simulink model "P414_1_model03_comp"  (R2021a)
settings: Solver=ode23tb  StartTime=0.0  StopTime=10  MaxStep=10/(60*24)  RelTol=1e-3
model workspace (MAT data in the model file):
  clima__A_c = 3295.16408265
  clima__A_f = 3100.53942116
  clima__G0 = [0.05; 0.00070738]
  clima__H = 7.9995824611
  clima__T0 = [287.15; 287.15; 287.15; 287.15]
  clima__T_ss = 280.150340169
  clima__alpha_c = 0.0100640347387
  clima__alpha_f = 0.0111385012129
  clima__alpha_i = 0.1
  clima__c_s = [1081 1081]
  clima__cd_c = 8736
  clima__d_c = 1.5
  clima__hour0 = 1
  clima__int_air_speed = 0.5
  clima__l_s = [0.1 0.1]
  clima__lam_s = [2.5 0.85]
  clima__minWindows = 0.299965865643
  clima__rhod_s = [2600 2500]
  clima__tau_c = 1
  crop__A_v = 2080
  crop__C = [0.01 0.001 0.01 0.01]
  crop__C_buf_max = 0.02
  crop__C_wv = 0.2
  crop__Chi_nutrients = [0.015625; 0.0104166666667; 0.00520833333333; 0.00208333333333; 0.00208333333333; 0.00104166666667; 0; 0]
  crop__N = [0; 0; 0; 0; 0; 0; 0; 0]
  crop__R = [0 0 0]
  crop__T_max_v = 40
  crop__T_max_v24 = 27
  crop__T_min_v = 6
  crop__T_min_v24 = 14
  crop__T_sum_end = 1035
  crop__T_v_start_fruit = 1100
  crop__Tsum = 0
  crop__Tv = 288
  crop__b_N_uptake = 0.5
  crop__c_fruit_g = 0.27
  crop__c_fruit_m = 2.3e-07
  crop__c_leaf_g = 0.28
  crop__c_leaf_m = 3.47e-07
  crop__c_stem_g = 0.3
  crop__c_stem_m = 1.47e-07
  crop__fraction_DM = 0.08
  crop__int_air_speed = 0.5
  crop__min_water_capacity = 0.1
  crop__plants_density = 2.1562
  crop__rg_fruit = 2e-07
  crop__rg_leaf = 9.5e-08
  crop__rg_stem = 7.4e-08
  crop__s_buforg_buf = -5000
  crop__s_max_T = 0.5793
  crop__s_max_T24 = 1.3904
  crop__s_min_T = -0.869
  crop__s_min_T24 = -1.1587
  heater__A_e = 0.0001
  heater__A_i = 0.008
  heater__T = 288
  heater__c = 5e-10
  heater__power = 60000000
  screen__Power = 100
  screen__Radthreshold = 900
  screen__beta = 2.23564167038e-14
  screen__gamma_max = 2.26308905438e-14
  screen__velocity = 0.333333333333
  subtrate__C_ws = 0.1
  subtrate__N = [0; 0; 0; 0; 0; 0; 0; 0]
  subtrate__Nmin_subs = 1e-09
  subtrate__Vmax_subs = 10
  subtrate__Vmin_subs = 0.01
  subtrate__sigma_max = 1
  subtrate__sigma_min = 1
  tomato__Cfruit0 = 0.001
  windows__AR = 19.9974923936
  windows__Power = 100
  windows__RadThreshold = 10
  windows__max_night = 10
  windows__tau = 600
values from neighbouring files (symbols this model uses):
  CO2_ppm_ext = 450    [P414_3_script_model03.m]    (also in P414_3_script_model03_compile.m = 400)
  maxvelocity = 1    [P414_3_script_model03.m]    (also in P414_3_script_model03_compile.m = 200)
  tend_crop1 = -days(t0-datetime('15-Aug-2022'))    [P414_3_script_model03.m]    (also in P414_3_script_model03_compile.m = 20)
  tend_crop2 = -days(t0-datetime('10-Dec-2022'))    [P414_3_script_model03.m]    (also in P414_3_script_model03_compile.m = 40)
  tinit_crop1 = -days(t0-datetime('16-Feb-2022'))    [P414_3_script_model03.m]    (also in P414_3_script_model03_compile.m = 1)
  tinit_crop2 = -days(t0-datetime('10-Jul-2022'))    [P414_3_script_model03.m]    (also in P414_3_script_model03_compile.m = 20)
  Tmax = 12 + 273.15    (= 285.15)    [P414_3_script_model03.m]
  today_days = floor(days(r.DateTime(end) - t0))    [P414_3_script_model03.m]    (also in P414_3_script_model03_compile.m = 5)
  Tstart = 9 + 273.15    (= 282.15)    [P414_3_script_model03.m]
  WinAR = 40    [P414_3_script_model03.m]    (also in P414_3_script_model03_compile.m = 10)
libraries: HORTISIM x15
settings Model: VariantFading=off  ParameterArgumentNames=clima__A_c,clima__A_f  OrderedModelArguments=off  Creator=djoroya  LastModifiedBy=djoroya
settings SolverCC: MaxConsecutiveMinStep=2
settings DataIOCC: SaveFormat=StructureWithTime
settings DebuggingCC: UnconnectedInputMsg=none  UnconnectedOutputMsg=none  UnconnectedLineMsg=none
settings HardwareCC: TargetBitPerLong=64  TargetBitPerPointer=64  TargetBitPerSizeT=64  TargetBitPerPtrDiffT=64  TargetLongLongMode=on  TargetIntDivRoundTo=Zero  TargetEndianess=LittleEndian  TargetWordSize=64  TargetHWDeviceType=MATLAB Host  ProdEqTarget=off
settings RTWCC: Description=Rapid Simulation Target  SystemTargetFile=rsim.tlc  TemplateMakefile=rsim_default_tmf
settings RSimTargetCC: TargetLangStandard=C99 (ISO)

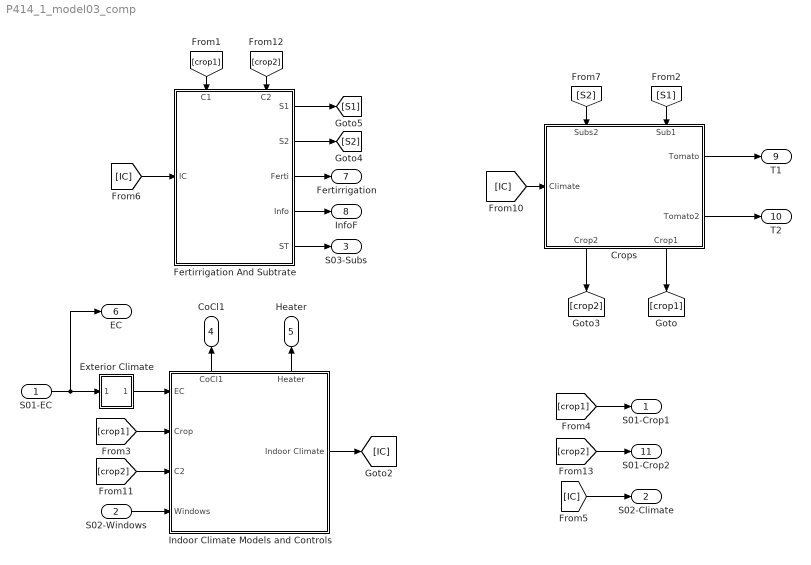
== system P414_1_model03_comp ==
  S01-EC : Inport
  S02-Windows : Inport  Port=2
  Crops : Subsystem
      settings: PortSchema="{\"entries\":[{\"content\":{\"sides\":[{\"content\":{\"connectorIds\":[\"In1\"]},\"type\":\"ConnectorPlacement.EquallySpacedRectSide\",\"uuid\":\"80596a6c-707e-446a-ab87-7a25f59fcc32\"},{\"content\":{\"connectorIds\":[\"Out1\",\"Out2\"],\"side\":\"RIGHT\"},\"type\":\"ConnectorPlacement.EquallySpacedRectSide\",\"uuid\":\"b8326ebd-de89-4eeb-b2a4-cbf566e8a818\"},{\"content\":{\"connectorIds\":[\"In2\",\"In3\"],\"side\":\"TOP\"},\"type\":\"ConnectorPlacement.EquallySpacedRectSide\",\"uuid\":\"5aa9e4b4-c649-4944-831f-92d2e7862f36\"},{\"content\":{\"connectorIds\":[\"Out3\",\"Out4\"],\"side\":\"BOTTOM\"},\"type\":\"ConnectorPlacement.EquallySpacedRectSide\",\"uuid\":\"3a07140b-9c77-4fd6-9860-89a6392cb8f1\"}]},\"type\":\"ConnectorPlacement.EquallySpacedConnector\",\"uuid\":\"ce31e92b-0c53-4f1c-a6e5-8defcbaa2f47\"}],\"packageUris\":[\"http://schema.mathworks.com/mf0/Connector/R2020b\"],\"version\":\"1.0\"}"
  Exterior Climate : Subsystem
  Fertirrigation And Subtrate : Subsystem
      settings: PortSchema="{\"entries\":[{\"content\":{\"sides\":[{\"content\":{\"connectorIds\":[\"In1\"]},\"type\":\"ConnectorPlacement.EquallySpacedRectSide\",\"uuid\":\"80596a6c-707e-446a-ab87-7a25f59fcc32\"},{\"content\":{\"connectorIds\":[\"Out1\",\"Out2\",\"Out3\",\"Out4\",\"Out5\"],\"side\":\"RIGHT\"},\"type\":\"ConnectorPlacement.EquallySpacedRectSide\",\"uuid\":\"b8326ebd-de89-4eeb-b2a4-cbf566e8a818\"},{\"content\":{\"connectorIds\":[\"In2\",\"In3\"],\"side\":\"TOP\"},\"type\":\"ConnectorPlacement.EquallySpacedRectSide\",\"uuid\":\"5aa9e4b4-c649-4944-831f-92d2e7862f36\"}]},\"type\":\"ConnectorPlacement.EquallySpacedConnector\",\"uuid\":\"ce31e92b-0c53-4f1c-a6e5-8defcbaa2f47\"}],\"packageUris\":[\"http://schema.mathworks.com/mf0/Connector/R2020b\"],\"version\":\"1.0\"}"
  Indoor Climate Models and Controls : Subsystem
      settings: PortSchema="{\"entries\":[{\"content\":{\"sides\":[{\"content\":{\"connectorIds\":[\"In1\",\"In2\",\"In3\",\"In4\"]},\"type\":\"ConnectorPlacement.EquallySpacedRectSide\",\"uuid\":\"f3cdb665-05cd-4c14-b99e-86a7cbd305f2\"},{\"content\":{\"connectorIds\":[\"Out1\"],\"side\":\"RIGHT\"},\"type\":\"ConnectorPlacement.EquallySpacedRectSide\",\"uuid\":\"ae9c6689-db0e-4adc-94c4-95f30f4a2385\"},{\"content\":{\"connectorIds\":[\"Out2\",\"Out3\"],\"side\":\"TOP\"},\"type\":\"ConnectorPlacement.EquallySpacedRectSide\",\"uuid\":\"b06e03f0-9ac9-40cc-8ad1-aa848145a491\"}]},\"type\":\"ConnectorPlacement.EquallySpacedConnector\",\"uuid\":\"03211f4f-961e-418c-be17-aa45c1620fb4\"}],\"packageUris\":[\"http://schema.mathworks.com/mf0/Connector/R2020b\"],\"version\":\"1.0\"}"
  S01-Crop1 : Outport
  S02-Climate : Outport  Port=2
  S03-Subs : Outport  Port=3
  CoCl1 : Outport  Port=4
  Heater : Outport  Port=5
  EC : Outport  Port=6
  Fertirrigation : Outport  Port=7
  InfoF : Outport  Port=8
  T1 : Outport  Port=9
  T2 : Outport  Port=10
  S01-Crop2 : Outport  Port=11
  wires:
  Exterior Climate/1(EC) -> Indoor Climate Models and Controls/1(EC)
  [crop1] -> Indoor Climate Models and Controls/2(Crop)
  S01-EC/1 -> EC/1, Exterior Climate/1(In1)
  [IC] -> S02-Climate/1
  [crop1] -> S01-Crop1/1
  Indoor Climate Models and Controls/2(CoCl1) -> CoCl1/1
  S02-Windows/1 -> Indoor Climate Models and Controls/4(Windows)
  Indoor Climate Models and Controls/3(Heater) -> Heater/1
  Indoor Climate Models and Controls/1(Indoor Climate) -> [IC]
  [crop1] -> Fertirrigation And Subtrate/2(C1)
  [crop2] -> Fertirrigation And Subtrate/3(C2)
  [IC] -> Fertirrigation And Subtrate/1(IC)
  Fertirrigation And Subtrate/1(S1) -> [S1]
  Fertirrigation And Subtrate/2(S2) -> [S2]
  Fertirrigation And Subtrate/3(Ferti) -> Fertirrigation/1
  Fertirrigation And Subtrate/4(Info) -> InfoF/1
  [crop2] -> Indoor Climate Models and Controls/3(C2)
  [crop2] -> S01-Crop2/1
  [S1] -> Crops/3(Sub1)
  [IC] -> Crops/1(Climate)
  [S2] -> Crops/2(Subs2)
  Crops/4(Crop1) -> [crop1]
  Crops/1(Tomato) -> T1/1
  Crops/3(Crop2) -> [crop2]
  Crops/2(Tomato2) -> T2/1
  Fertirrigation And Subtrate/5(ST) -> S03-Subs/1

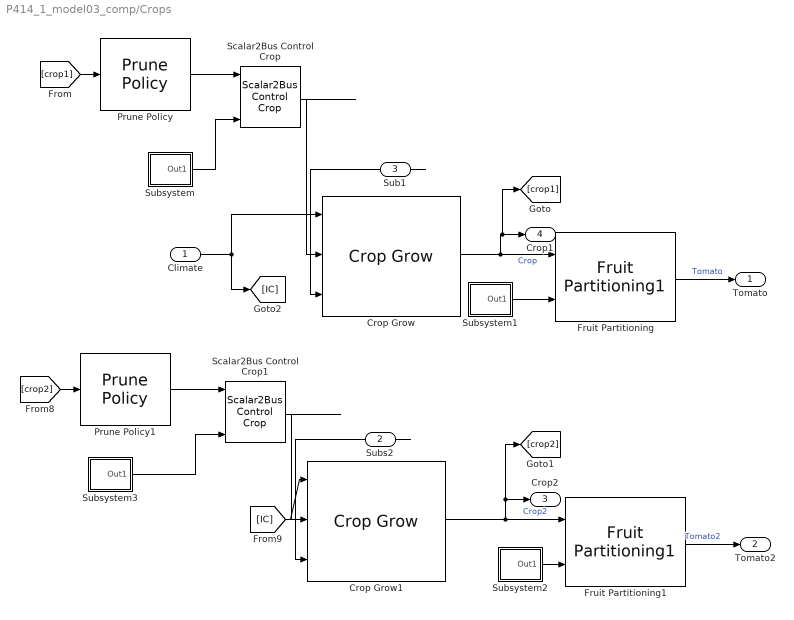
== system P414_1_model03_comp/Crops ==
  Climate : Inport
  Subs2 : Inport  Port=2
  Sub1 : Inport  Port=3
  Crop Grow : HORTISIM/Horticulture/Models/Crop Grow  Chi_nutrients=crop__Chi_nutrients  A_v=crop__A_v  plants_density=crop__plants_density  fraction_DM=crop__fraction_DM  min_water_capacity=crop__min_water_capacity  C_buf_max=crop__C_buf_max  T_v_start_fruit=crop__T_v_start_fruit  int_air_speed=crop__int_air_speed  b_N_uptake=crop__b_N_uptake  Tv=crop__Tv  C=crop__C  R=crop__R  Tsum=crop__Tsum  C_wv=crop__C_wv  N=crop__N  rg_fruit=crop__rg_fruit  c_fruit_m=crop__c_fruit_m  c_fruit_g=crop__c_fruit_g  rg_leaf=crop__rg_leaf  c_leaf_m=crop__c_leaf_m  c_leaf_g=crop__c_leaf_g  rg_stem=crop__rg_stem  c_stem_m=crop__c_stem_m  c_stem_g=crop__c_stem_g  VelocityAbsortion=crop__VelocityAbsortion  T_max_v=crop__T_max_v  s_max_T=crop__s_max_T  s_min_T=crop__s_min_T  s_buforg_buf=crop__s_buforg_buf  T_sum_end=crop__T_sum_end  T_max_v24=crop__T_max_v24  T_min_v24=crop__T_min_v24  s_min_T24=crop__s_min_T24  s_max_T24=crop__s_max_T24  T_min_v=crop__T_min_v
      settings: SourceProductName=Horti Simulator
  Crop Grow1 : HORTISIM/Horticulture/Models/Crop Grow  Chi_nutrients=crop__Chi_nutrients  A_v=crop__A_v  plants_density=crop__plants_density  fraction_DM=crop__fraction_DM  min_water_capacity=crop__min_water_capacity  C_buf_max=crop__C_buf_max  T_v_start_fruit=crop__T_v_start_fruit  int_air_speed=crop__int_air_speed  b_N_uptake=crop__b_N_uptake  Tv=crop__Tv  C=crop__C  R=crop__R  Tsum=crop__Tsum  C_wv=crop__C_wv  N=crop__N  rg_fruit=crop__rg_fruit  c_fruit_m=crop__c_fruit_m  c_fruit_g=crop__c_fruit_g  rg_leaf=crop__rg_leaf  c_leaf_m=crop__c_leaf_m  c_leaf_g=crop__c_leaf_g  rg_stem=crop__rg_stem  c_stem_m=crop__c_stem_m  c_stem_g=crop__c_stem_g  VelocityAbsortion=crop__VelocityAbsortion  T_max_v=crop__T_max_v  s_max_T=crop__s_max_T  s_min_T=crop__s_min_T  s_buforg_buf=crop__s_buforg_buf  T_sum_end=crop__T_sum_end  T_max_v24=crop__T_max_v24  T_min_v24=crop__T_min_v24  s_min_T24=crop__s_min_T24  s_max_T24=crop__s_max_T24  T_min_v=crop__T_min_v
      settings: SourceProductName=Horti Simulator
  Fruit Partitioning : HORTISIM/Horticulture/Models/Fruit Partitioning1  Cfruit0=1e-3
      settings: SourceProductName=Horti Simulator
  Fruit Partitioning1 : HORTISIM/Horticulture/Models/Fruit Partitioning1  Cfruit0=tomato__Cfruit0
      settings: SourceProductName=Horti Simulator
  Prune Policy : HORTISIM/Horticulture/Controls/Prune Policy  SystemSampleTime=-1  VariantActivationTime=update diagram  Latency=0  AutoFrameSizeCalculation=off
      settings: SourceProductName=Horti Simulator
  Prune Policy1 : HORTISIM/Horticulture/Controls/Prune Policy  SystemSampleTime=-1  VariantActivationTime=update diagram  Latency=0  AutoFrameSizeCalculation=off
      settings: SourceProductName=Horti Simulator
  Scalar2Bus Control Crop : HORTISIM/Other  Functions/Scalar2Bus Control Crop  SystemSampleTime=-1  VariantActivationTime=update diagram  Latency=0  AutoFrameSizeCalculation=off
      settings: SourceProductName=Horti Simulator
  Scalar2Bus Control Crop1 : HORTISIM/Other  Functions/Scalar2Bus Control Crop  SystemSampleTime=-1  VariantActivationTime=update diagram  Latency=0  AutoFrameSizeCalculation=off
      settings: SourceProductName=Horti Simulator
  Subsystem : Subsystem  mask{tinit=tinit_crop1, tend=tend_crop1}
  Subsystem1 : Subsystem  mask{tinit=tinit_crop1, tend=tend_crop1}
  Subsystem2 : Subsystem  mask{tinit=tinit_crop2, tend=tend_crop2}
  Subsystem3 : Subsystem  mask{tinit=tinit_crop2, tend=tend_crop2}
  Tomato : Outport
  Tomato2 : Outport  Port=2
  Crop2 : Outport  Port=3
  Crop1 : Outport  Port=4
  wires:
  Subs2/1 -> Crop Grow1/3
  Fruit Partitioning/1 -> Tomato/1  "Tomato"
  Scalar2Bus Control Crop1/1 -> Crop Grow1/2
  Sub1/1 -> Crop Grow/3
  Subsystem/1(Out1) -> Scalar2Bus Control Crop/4
  [IC] -> Crop Grow1/1
  [crop2] -> Prune Policy1/1
  Crop Grow1/1 -> [crop2], Crop2/1, Fruit Partitioning1/1  "Crop2"
  Fruit Partitioning1/1 -> Tomato2/1  "Tomato2"
  Subsystem1/1(Out1) -> Fruit Partitioning/2
  Prune Policy/1 -> Scalar2Bus Control Crop/1
  Subsystem2/1(Out1) -> Fruit Partitioning1/2
  [crop1] -> Prune Policy/1
  Subsystem3/1(Out1) -> Scalar2Bus Control Crop1/4
  Crop Grow/1 -> [crop1], Crop1/1, Fruit Partitioning/1  "Crop"
  Scalar2Bus Control Crop/1 -> Crop Grow/2
  Climate/1 -> [IC], Crop Grow/1
  Prune Policy1/1 -> Scalar2Bus Control Crop1/1

== system P414_1_model03_comp/Exterior Climate ==
  In1 : Inport
  CO2 ppm : Constant  Value=CO2_ppm_ext
  Demux : Demux
  Scalar2Bus Exterior Climate : Subsystem
  EC : Outport
  wires:
  Demux/3 -> Scalar2Bus Exterior Climate/3(Wind)
  Demux/2 -> Scalar2Bus Exterior Climate/2(Radiation)
  Scalar2Bus Exterior Climate/1(EC) -> EC/1
  Demux/1 -> Scalar2Bus Exterior Climate/1(Temperature)
  Demux/4 -> Scalar2Bus Exterior Climate/4(Humidity)
  In1/1 -> Demux/1
  CO2 ppm/1 -> Scalar2Bus Exterior Climate/5(CO2)

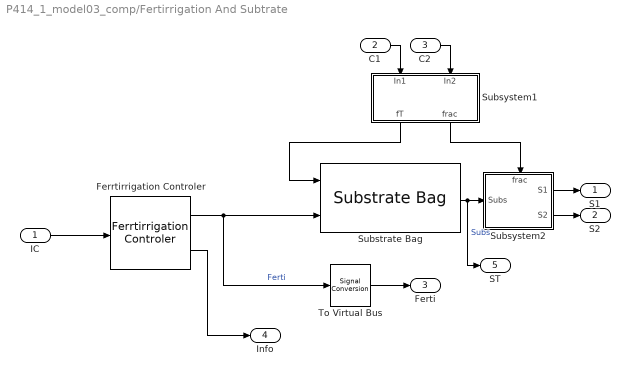
== system P414_1_model03_comp/Fertirrigation And Subtrate ==
  IC : Inport
  C1 : Inport  Port=2
  C2 : Inport  Port=3
  Ferrtirrigation Controler : HORTISIM/Horticulture/Controls/Ferrtirrigation  Controler  hour0=irrigation__hour0  IrrigationFlow=irrigation__IrrigationFlow  Xnutrients=irrigation__Xnutrients  percent_irrigation=irrigation__percent_irrigation  Irrigation_jules_to_hours=irrigation__Irrigation_jules_to_hours
      settings: SourceProductName=Horti Simulator
  Substrate Bag : HORTISIM/Horticulture/Models/Substrate Bag  Vmax_subs=subtrate__Vmax_subs  Vmin_subs=subtrate__Vmin_subs  Nmin_subs=subtrate__Nmin_subs  C_ws=subtrate__C_ws  N=subtrate__N  DraingeConst=subtrate__DraingeConst  sigma_max=subtrate__sigma_max  sigma_min=subtrate__sigma_min
      settings: SourceProductName=Horti Simulator
  Subsystem1 : Subsystem
  Subsystem2 : Subsystem
      settings: PortSchema="{\"entries\":[{\"content\":{\"sides\":[{\"content\":{\"connectorIds\":[\"In1\"]},\"type\":\"ConnectorPlacement.EquallySpacedRectSide\",\"uuid\":\"526c2ba0-7984-4a67-b75e-815cf79b4473\"},{\"content\":{\"connectorIds\":[\"Out1\",\"Out2\"],\"side\":\"RIGHT\"},\"type\":\"ConnectorPlacement.EquallySpacedRectSide\",\"uuid\":\"1f428ce7-4be7-4b4c-9b6b-ebbf12a2ebe7\"},{\"content\":{\"connectorIds\":[\"In2\"],\"side\":\"TOP\"},\"type\":\"ConnectorPlacement.EquallySpacedRectSide\",\"uuid\":\"5866ee80-50d2-4205-943e-212db577b0a0\"}]},\"type\":\"ConnectorPlacement.EquallySpacedConnector\",\"uuid\":\"0f7aadc1-005b-462a-894f-416c66164dac\"}],\"packageUris\":[\"http://schema.mathworks.com/mf0/Connector/R2020b\"],\"version\":\"1.0\"}"
  To Virtual Bus : SignalConversion  ConversionOutput=Virtual bus  OverrideOpt=off
  S1 : Outport
  S2 : Outport  Port=2
  Ferti : Outport  Port=3
  Info : Outport  Port=4
  ST : Outport  Port=5
  wires:
  C2/1 -> Subsystem1/2(In2)
  Subsystem1/2(frac) -> Subsystem2/2(frac)
  Ferrtirrigation Controler/1 -> Substrate Bag/2, To Virtual Bus/1  "Ferti"
  Subsystem2/1(S1) -> S1/1
  C1/1 -> Subsystem1/1(In1)
  Ferrtirrigation Controler/2 -> Info/1
  Subsystem2/2(S2) -> S2/1
  IC/1 -> Ferrtirrigation Controler/1
  To Virtual Bus/1 -> Ferti/1
  Substrate Bag/1 -> ST/1, Subsystem2/1(Subs)  "Subs"
  Subsystem1/1(fT) -> Substrate Bag/1

== system P414_1_model03_comp/Indoor Climate Models and Controls ==
  EC : Inport
  Crop : Inport  Port=2
  C2 : Inport  Port=3
  Windows : Inport  Port=4
  Climate Model : HORTISIM/Climate/Models/Climate Model  hour0=clima__hour0  G0=clima__G0  T0=clima__T0  H=clima__H  A_f=clima__A_f  A_c=clima__A_c  minWindows=clima__minWindows  lam_s=clima__lam_s  c_s=clima__c_s  l_s=clima__l_s  rhod_s=clima__rhod_s  int_air_speed=clima__int_air_speed  alpha_i=clima__alpha_i  alpha_c=clima__alpha_c  tau_c=clima__tau_c  alpha_f=clima__alpha_f  d_c=clima__d_c  cd_c=clima__cd_c  T_ss=clima__T_ss
      settings: SourceProductName=Horti Simulator
  Control System : Subsystem
      settings: PortSchema="{\"entries\":[{\"content\":{\"sides\":[{\"content\":{\"connectorIds\":[\"In1\",\"In2\",\"In3\",\"In4\"]},\"type\":\"ConnectorPlacement.EquallySpacedRectSide\",\"uuid\":\"7d0146e2-a53b-49ab-a7f4-04cd7ef00b9a\"},{\"content\":{\"connectorIds\":[\"Out1\",\"Out2\"],\"side\":\"RIGHT\"},\"type\":\"ConnectorPlacement.EquallySpacedRectSide\",\"uuid\":\"fee587e2-4b5c-4140-8904-07609d427593\"},{\"content\":{\"connectorIds\":[],\"side\":\"TOP\"},\"type\":\"ConnectorPlacement.EquallySpacedRectSide\",\"uuid\":\"52e767bc-1595-40ac-996f-44c9eedd0a08\"},{\"content\":{\"connectorIds\":[\"Out3\",\"In5\"],\"side\":\"BOTTOM\"},\"type\":\"ConnectorPlacement.EquallySpacedRectSide\",\"uuid\":\"c629db5c-cfe6-4bd1-aeb9-7fba46dde396\"}]},\"type\":\"ConnectorPlacement.EquallySpacedConnector\",\"uuid\":\"268fde01-3c08-4d62-bfbb-fc94284c5cdd\"}],\"packageUris\":[\"http://schema.mathworks.com/mf0/Connector/R2020b\"],\"version\":\"1.0\"}"
  Indoor Climate : Outport
  CoCl1 : Outport  Port=2
  Heater : Outport  Port=3
  wires:
  Climate Model/1 -> Control System/2(IC), Indoor Climate/1  "Indoor Climate"
  Control System/2(CoCl1) -> Climate Model/2, CoCl1/1  "Control"
  Control System/1(Ext) -> Climate Model/1
  EC/1 -> Climate Model/3, Control System/5(EC)
  Crop/1 -> Control System/3(C1)
  Windows/1 -> Control System/1(Windows)
  Control System/3(Heater) -> Heater/1
  C2/1 -> Control System/4(C2)

== system P414_1_model03_comp/Crops/Subsystem ==
  Clock : Clock
  Constant : Constant  Value=tinit
  Constant1 : Constant  Value=tend
  If : If  NumInputs=3  IfExpression=(u1>u2)&(u1<u3)
  If Action Subsystem : Subsystem  TreatAsAtomicUnit=on
  If Action Subsystem1 : Subsystem  TreatAsAtomicUnit=on
  Merge : Merge
  Out1 : Outport
  wires:
  Clock/1 -> If/1
  Constant/1 -> If/2
  Constant1/1 -> If/3
  If/1 -> If Action Subsystem/Action
  If/2 -> If Action Subsystem1/Action
  If Action Subsystem/1(Out1) -> Merge/1
  If Action Subsystem1/1(Out1) -> Merge/2
  Merge/1 -> Out1/1

== system P414_1_model03_comp/Crops/Subsystem1 ==
  Clock : Clock
  Constant : Constant  Value=tinit
  Constant1 : Constant  Value=tend
  If : If  NumInputs=3  IfExpression=(u1>u2)&(u1<u3)
  If Action Subsystem : Subsystem  TreatAsAtomicUnit=on
  If Action Subsystem1 : Subsystem  TreatAsAtomicUnit=on
  Merge : Merge
  Out1 : Outport
  wires:
  Clock/1 -> If/1
  Constant/1 -> If/2
  Constant1/1 -> If/3
  If/1 -> If Action Subsystem/Action
  If/2 -> If Action Subsystem1/Action
  If Action Subsystem/1(Out1) -> Merge/1
  If Action Subsystem1/1(Out1) -> Merge/2
  Merge/1 -> Out1/1

== system P414_1_model03_comp/Crops/Subsystem2 ==
  Clock : Clock
  Constant : Constant  Value=tinit
  Constant1 : Constant  Value=tend
  If : If  NumInputs=3  IfExpression=(u1>u2)&(u1<u3)
  If Action Subsystem : Subsystem  TreatAsAtomicUnit=on
  If Action Subsystem1 : Subsystem  TreatAsAtomicUnit=on
  Merge : Merge
  Out1 : Outport
  wires:
  Clock/1 -> If/1
  Constant/1 -> If/2
  Constant1/1 -> If/3
  If/1 -> If Action Subsystem/Action
  If/2 -> If Action Subsystem1/Action
  If Action Subsystem/1(Out1) -> Merge/1
  If Action Subsystem1/1(Out1) -> Merge/2
  Merge/1 -> Out1/1

== system P414_1_model03_comp/Crops/Subsystem3 ==
  Clock : Clock
  Constant : Constant  Value=tinit
  Constant1 : Constant  Value=tend
  If : If  NumInputs=3  IfExpression=(u1>u2)&(u1<u3)
  If Action Subsystem : Subsystem  TreatAsAtomicUnit=on
  If Action Subsystem1 : Subsystem  TreatAsAtomicUnit=on
  Merge : Merge
  Out1 : Outport
  wires:
  Clock/1 -> If/1
  Constant/1 -> If/2
  Constant1/1 -> If/3
  If/1 -> If Action Subsystem/Action
  If/2 -> If Action Subsystem1/Action
  If Action Subsystem/1(Out1) -> Merge/1
  If Action Subsystem1/1(Out1) -> Merge/2
  Merge/1 -> Out1/1

== system P414_1_model03_comp/Exterior Climate/Scalar2Bus Exterior Climate ==
  Temperature : Inport
  Radiation : Inport  Port=2
  Wind : Inport  Port=3
  Humidity : Inport  Port=4
  CO2 : Inport  Port=5
  Bus Creator : BusCreator  Inputs=5
  EC : Outport
  wires:
  Humidity/1 -> Bus Creator/3  "HR"
  Wind/1 -> Bus Creator/4  "Wind"
  Temperature/1 -> Bus Creator/1  "Temp"
  Bus Creator/1 -> EC/1
  Radiation/1 -> Bus Creator/2  "Rad"
  CO2/1 -> Bus Creator/5  "Cppm"

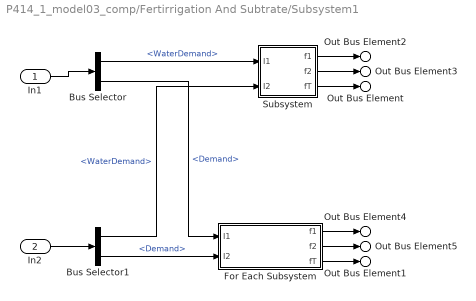
== system P414_1_model03_comp/Fertirrigation And Subtrate/Subsystem1 ==
  In1 : Inport
  In2 : Inport  Port=2
  Bus Selector : BusSelector  OutputSignals=Water.WaterFlows.WaterDemand,Nutrients.Demand
  Bus Selector1 : BusSelector  OutputSignals=Water.WaterFlows.WaterDemand,Nutrients.Demand
  For Each Subsystem : Subsystem  TreatAsAtomicUnit=on
  Subsystem : Subsystem
  Out Bus Element1 : Outport  PortName=fT  Element=Nutrients.Demand
  Out Bus Element : Outport  PortName=fT  Element=Water.WaterFlows.WaterDemand
  Out Bus Element2 : Outport  Port=2  PortName=frac  Element=water.f1
  Out Bus Element3 : Outport  Port=2  PortName=frac  Element=water.f2
  Out Bus Element4 : Outport  Port=2  PortName=frac  Element=nutrients.f1
  Out Bus Element5 : Outport  Port=2  PortName=frac  Element=nutrients.f2
  wires:
  In1/1 -> Bus Selector/1
  In2/1 -> Bus Selector1/1
  Bus Selector1/1 -> Subsystem/2(I2)  "<WaterDemand>"
  Bus Selector/1 -> Subsystem/1(I1)  "<WaterDemand>"
  Subsystem/3(fT) -> Out Bus Element/1
  Subsystem/1(f1) -> Out Bus Element2/1
  Subsystem/2(f2) -> Out Bus Element3/1
  Bus Selector/2 -> For Each Subsystem/1(I1)  "<Demand>"
  Bus Selector1/2 -> For Each Subsystem/2(I2)  "<Demand>"
  For Each Subsystem/3(fT) -> Out Bus Element1/1
  For Each Subsystem/2(f2) -> Out Bus Element5/1
  For Each Subsystem/1(f1) -> Out Bus Element4/1

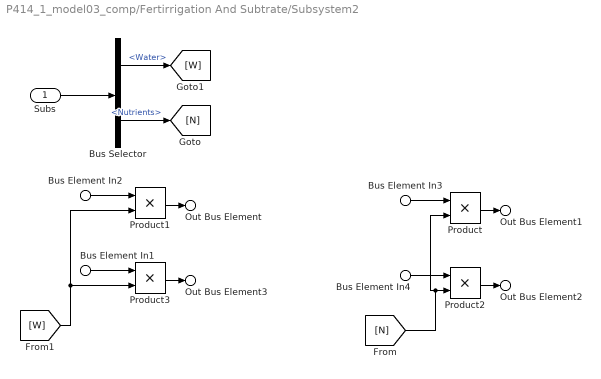
== system P414_1_model03_comp/Fertirrigation And Subtrate/Subsystem2 ==
  Subs : Inport
  Bus Element In2 : Inport  Port=2  PortName=frac  Element=water.f1
  Bus Element In1 : Inport  Port=2  PortName=frac  Element=water.f2
  Bus Element In3 : Inport  Port=2  PortName=frac  Element=nutrients.f1
  Bus Element In4 : Inport  Port=2  PortName=frac  Element=nutrients.f2
  Bus Selector : BusSelector  OutputSignals=Uptake.Water,Uptake.Nutrients
  Product{,1..3} (4 alike) : Product
  Out Bus Element : Outport  PortName=S1  Element=Uptake.Water
  Out Bus Element1 : Outport  PortName=S1  Element=Uptake.Nutrients
  Out Bus Element3 : Outport  Port=2  PortName=S2  Element=Uptake.Water
  Out Bus Element2 : Outport  Port=2  PortName=S2  Element=Uptake.Nutrients
  wires:
  Subs/1 -> Bus Selector/1
  Bus Selector/1 -> [W]  "<Water>"
  Bus Selector/2 -> [N]  "<Nutrients>"
  Bus Element In3/1 -> Product/1
  Bus Element In2/1 -> Product1/1
  Bus Element In4/1 -> Product2/1
  [N] -> Product/2, Product2/2
  Bus Element In1/1 -> Product3/1
  [W] -> Product3/2, Product1/2
  Product1/1 -> Out Bus Element/1
  Product3/1 -> Out Bus Element3/1
  Product/1 -> Out Bus Element1/1
  Product2/1 -> Out Bus Element2/1

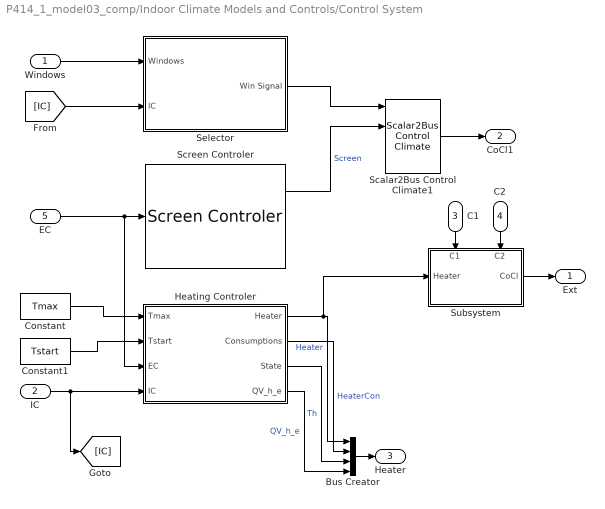
== system P414_1_model03_comp/Indoor Climate Models and Controls/Control System ==
  Windows : Inport
  IC : Inport  Port=2
  C1 : Inport  Port=3
  C2 : Inport  Port=4
  EC : Inport  Port=5
  Bus Creator : BusCreator  Inputs=4
  Constant : Constant  Value=Tmax
  Constant1 : Constant  Value=Tstart
  Heating Controler : Subsystem  AncestorBlock=HORTISIM/Climate/Controls/Heating Controler  mask{T=heater__T, power=heater__power, A_e=heater__A_e, A_i=heater__A_i, c=heater__c}
      mask DialogControl InitialCondition Prompt: Initial Condition
      mask DialogControl Parameters Prompt: Parameters
      mask Display: image('$imagefile'); % Use "Edit Image" on toolstrip to change.
  Scalar2Bus Control Climate1 : HORTISIM/Other  Functions/Scalar2Bus  Control Climate  SystemSampleTime=-1  VariantActivationTime=update diagram  Latency=0  AutoFrameSizeCalculation=off
      settings: SourceProductName=Horti Simulator
  Screen Controler : HORTISIM/Climate/Controls/Screen Controler  Radthreshold=200  velocity=0.33333  Power=0  gamma_max=0.3  beta=0.1
      settings: SourceProductName=Horti Simulator
  Selector : Subsystem
  Subsystem : Subsystem
      settings: PortSchema="{\"entries\":[{\"content\":{\"sides\":[{\"content\":{\"connectorIds\":[\"In1\"]},\"type\":\"ConnectorPlacement.EquallySpacedRectSide\",\"uuid\":\"d19974ff-f02b-4de0-b9d2-af7ff1541749\"},{\"content\":{\"connectorIds\":[\"Out1\"],\"side\":\"RIGHT\"},\"type\":\"ConnectorPlacement.EquallySpacedRectSide\",\"uuid\":\"996386bc-d441-4074-8822-a847efaf7161\"},{\"content\":{\"connectorIds\":[\"In2\",\"In3\"],\"side\":\"TOP\"},\"type\":\"ConnectorPlacement.EquallySpacedRectSide\",\"uuid\":\"19980254-f226-445c-8822-1dc223142f79\"}]},\"type\":\"ConnectorPlacement.EquallySpacedConnector\",\"uuid\":\"a52359a0-275e-4596-8c51-69b7f984311f\"}],\"packageUris\":[\"http://schema.mathworks.com/mf0/Connector/R2020b\"],\"version\":\"1.0\"}"
  Ext : Outport
  CoCl1 : Outport  Port=2
  Heater : Outport  Port=3
  wires:
  EC/1 -> Heating Controler/3(EC), Screen Controler/1
  Constant1/1 -> Heating Controler/2(Tstart)
  Constant/1 -> Heating Controler/1(Tmax)
  Scalar2Bus Control Climate1/1 -> CoCl1/1
  Screen Controler/1 -> Scalar2Bus Control Climate1/2  "Screen"
  IC/1 -> [IC], Heating Controler/4(IC)
  Heating Controler/1(Heater) -> Subsystem/1(Heater), Bus Creator/1  "Heater"
  Heating Controler/2(Consumptions) -> Bus Creator/2  "HeaterCon"
  Heating Controler/3(State) -> Bus Creator/3  "Th"
  Bus Creator/1 -> Heater/1
  Windows/1 -> Selector/1(Windows)
  Selector/1(Win Signal) -> Scalar2Bus Control Climate1/1
  [IC] -> Selector/2(IC)
  Heating Controler/4(QV_h_e) -> Bus Creator/4  "QV_h_e"
  C2/1 -> Subsystem/3(C2)
  C1/1 -> Subsystem/2(C1)
  Subsystem/1(CoCl) -> Ext/1

== system P414_1_model03_comp/Crops/Subsystem/If Action Subsystem ==
  Action Port : ActionPort  ActionPortLabel=if((u1>u2)&(u1<u3))
  Constant : Constant
  Out1 : Outport
  wires:
  Constant/1 -> Out1/1

== system P414_1_model03_comp/Crops/Subsystem/If Action Subsystem1 ==
  Action Port : ActionPort  ActionPortLabel=else
  Constant : Constant  Value=0
  Out1 : Outport
  wires:
  Constant/1 -> Out1/1

== system P414_1_model03_comp/Crops/Subsystem1/If Action Subsystem ==
  Action Port : ActionPort  ActionPortLabel=if((u1>u2)&(u1<u3))
  Constant : Constant
  Out1 : Outport
  wires:
  Constant/1 -> Out1/1

== system P414_1_model03_comp/Crops/Subsystem1/If Action Subsystem1 ==
  Action Port : ActionPort  ActionPortLabel=else
  Constant : Constant  Value=0
  Out1 : Outport
  wires:
  Constant/1 -> Out1/1

== system P414_1_model03_comp/Crops/Subsystem2/If Action Subsystem ==
  Action Port : ActionPort  ActionPortLabel=if((u1>u2)&(u1<u3))
  Constant : Constant
  Out1 : Outport
  wires:
  Constant/1 -> Out1/1

== system P414_1_model03_comp/Crops/Subsystem2/If Action Subsystem1 ==
  Action Port : ActionPort  ActionPortLabel=else
  Constant : Constant  Value=0
  Out1 : Outport
  wires:
  Constant/1 -> Out1/1

== system P414_1_model03_comp/Crops/Subsystem3/If Action Subsystem ==
  Action Port : ActionPort  ActionPortLabel=if((u1>u2)&(u1<u3))
  Constant : Constant
  Out1 : Outport
  wires:
  Constant/1 -> Out1/1

== system P414_1_model03_comp/Crops/Subsystem3/If Action Subsystem1 ==
  Action Port : ActionPort  ActionPortLabel=else
  Constant : Constant  Value=0
  Out1 : Outport
  wires:
  Constant/1 -> Out1/1

== system P414_1_model03_comp/Fertirrigation And Subtrate/Subsystem1/For Each Subsystem ==
  I1 : Inport  Partition=on  PartitionDimension=1  PartitionWidth=1  PartitionOffset=0
  I2 : Inport  Port=2  Partition=on  PartitionDimension=1  PartitionWidth=1  PartitionOffset=0
  For Each : ForEach  DisableCoverage=on
  Subsystem : Subsystem
  f1 : Outport  ConcatenationDimension=1
  f2 : Outport  Port=2  ConcatenationDimension=1
  fT : Outport  Port=3  ConcatenationDimension=1
  wires:
  I2/1 -> Subsystem/2(I2)
  I1/1 -> Subsystem/1(I1)
  Subsystem/3(fT) -> fT/1
  Subsystem/2(f2) -> f2/1
  Subsystem/1(f1) -> f1/1

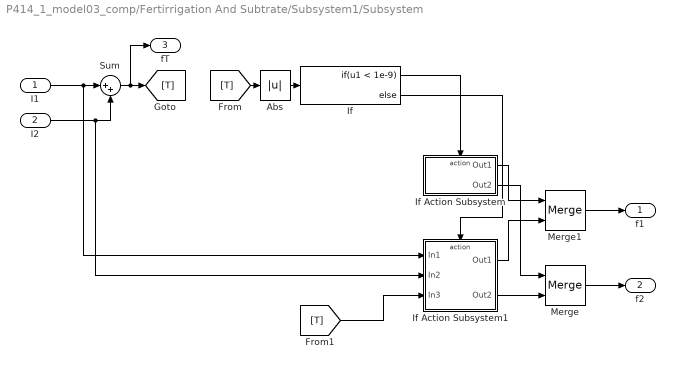
== system P414_1_model03_comp/Fertirrigation And Subtrate/Subsystem1/Subsystem ==
  I1 : Inport
  I2 : Inport  Port=2
  Abs : Abs  ZeroCross=off
  If : If  IfExpression=u1 < 1e-9  ZeroCross=off
  If Action Subsystem : Subsystem  TreatAsAtomicUnit=on
  If Action Subsystem1 : Subsystem  TreatAsAtomicUnit=on
  Merge : Merge
  Merge1 : Merge
  Sum : Sum  Inputs=|++
  f1 : Outport
  f2 : Outport  Port=2
  fT : Outport  Port=3
  wires:
  I1/1 -> If Action Subsystem1/1(In1), Sum/1
  I2/1 -> If Action Subsystem1/2(In2), Sum/2
  Sum/1 -> fT/1, [T]
  If/1 -> If Action Subsystem/Action
  If/2 -> If Action Subsystem1/Action
  [T] -> If Action Subsystem1/3(In3)
  If Action Subsystem/2(Out2) -> Merge/1
  If Action Subsystem1/2(Out2) -> Merge/2
  Merge/1 -> f2/1
  Merge1/1 -> f1/1
  If Action Subsystem1/1(Out1) -> Merge1/2
  If Action Subsystem/1(Out1) -> Merge1/1
  Abs/1 -> If/1
  [T] -> Abs/1

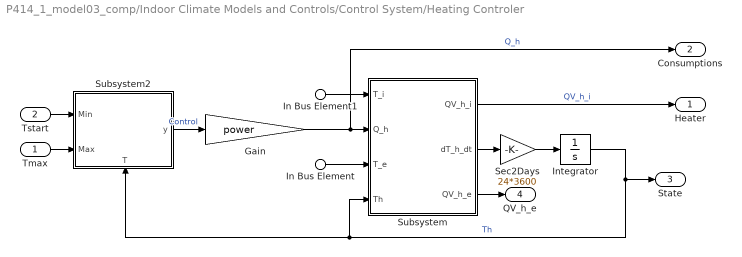
== system P414_1_model03_comp/Indoor Climate Models and Controls/Control System/Heating Controler ==
  Tmax : Inport
  Tstart : Inport  Port=2
  In Bus Element : Inport  Port=3  PortName=EC  Element=Temp
  In Bus Element1 : Inport  Port=4  PortName=IC  Element=Temp.Tair
  Gain : Gain  Gain=power
  Integrator : Integrator  InitialCondition=T  AbsoluteTolerance=0.001
  Sec2Days : Gain  Gain=24*3600
  Subsystem : Subsystem
  Subsystem2 : Subsystem
      settings: PortSchema="{\"entries\":[{\"content\":{\"sides\":[{\"content\":{\"connectorIds\":[\"In1\",\"In2\"]},\"type\":\"ConnectorPlacement.EquallySpacedRectSide\",\"uuid\":\"76a0539e-cd8b-47df-82d9-61971d3be914\"},{\"content\":{\"connectorIds\":[\"Out1\"],\"side\":\"RIGHT\"},\"type\":\"ConnectorPlacement.EquallySpacedRectSide\",\"uuid\":\"93f2ebb7-6ab4-4fcc-bc7a-3583f1db6e8e\"},{\"content\":{\"connectorIds\":[],\"side\":\"TOP\"},\"type\":\"ConnectorPlacement.EquallySpacedRectSide\",\"uuid\":\"b50a0ff6-3876-4dcb-8bb9-79340929aa80\"},{\"content\":{\"connectorIds\":[\"In3\"],\"side\":\"BOTTOM\"},\"type\":\"ConnectorPlacement.EquallySpacedRectSide\",\"uuid\":\"63f2a7a5-83ef-48e2-af90-7d61b47411e6\"}]},\"type\":\"ConnectorPlacement.EquallySpacedConnector\",\"uuid\":\"d97900b9-3143-4b55-b66d-f73dd0302926\"}],\"packageUris\":[\"http://schema.mathworks.com/mf0/Connector/R2020b\"],\"version\":\"1.0\"}"
  Heater : Outport  Unit=J
  Consumptions : Outport  Port=2
  State : Outport  Port=3
  QV_h_e : Outport  Port=4
  wires:
  Gain/1 -> Consumptions/1, Subsystem/2(Q_h)  "Q_h"
  Tstart/1 -> Subsystem2/1(" Min")
  Tmax/1 -> Subsystem2/2(Max)
  Subsystem2/1(y) -> Gain/1  "Control"
  Sec2Days/1 -> Integrator/1
  In Bus Element1/1 -> Subsystem/1(T_i)
  In Bus Element/1 -> Subsystem/3(T_e)
  Subsystem/1(QV_h_i) -> Heater/1  "QV_h_i"
  Subsystem/2(dT_h_dt) -> Sec2Days/1
  Integrator/1 -> State/1, Subsystem/4(Th), Subsystem2/3(T)  "Th"
  Subsystem/3(QV_h_e) -> QV_h_e/1

== system P414_1_model03_comp/Indoor Climate Models and Controls/Control System/Selector ==
  Windows : Inport
  IC : Inport  Port=2
  Bus Creator : BusCreator  Inputs=2
  Bus Selector : BusSelector  OutputSignals=value,AR
  Clock : Clock
  Constant3 : Constant  Value=today_days
  If : If  NumInputs=2  IfExpression=u2 > u1
  If Action Subsystem : Subsystem  TreatAsAtomicUnit=on
  If Action Subsystem1 : Subsystem  TreatAsAtomicUnit=on
  Merge : Merge
  Rate Limiter : RateLimiter  RisingSlewLimit=maxvelocity*60*24  FallingSlewLimit=-maxvelocity*60*24  SampleTimeMode=inherited
  Win Signal : Outport
  wires:
  If/2 -> If Action Subsystem/Action
  Windows/1 -> If Action Subsystem/1(Windows)
  If Action Subsystem1/1(Out1) -> Merge/1
  IC/1 -> If Action Subsystem1/1(In1)
  If Action Subsystem/1(Out1) -> Merge/2
  If/1 -> If Action Subsystem1/Action
  Clock/1 -> If/2
  Constant3/1 -> If/1
  Bus Creator/1 -> Win Signal/1
  Merge/1 -> Bus Selector/1
  Bus Selector/2 -> Bus Creator/2  "<AR>"
  Bus Selector/1 -> Rate Limiter/1  "<value>"
  Rate Limiter/1 -> Bus Creator/1  "value"

== system P414_1_model03_comp/Indoor Climate Models and Controls/Control System/Subsystem ==
  Heater : Inport
  C1 : Inport  Port=2
  C2 : Inport  Port=3
  Bus Selector : BusSelector  OutputSignals=HeatVars.QV,HeatVars.QT,A_v,CC
  Bus Selector1 : BusSelector  OutputSignals=HeatVars.QV,HeatVars.QT,CC
  "Scalar2Bus " : Subsystem
  Sum : Sum  Inputs=+++
  Sum1 : Sum  Inputs=++|
  Sum2 : Sum  Inputs=++|
  CoCl : Outport
  wires:
  C1/1 -> Bus Selector/1
  C2/1 -> Bus Selector1/1
  Bus Selector/4 -> Sum2/2  "<CC>"
  Sum/1 -> "Scalar2Bus "/1(QV)
  Sum1/1 -> "Scalar2Bus "/2(QT)
  Bus Selector/1 -> Sum/3  "<QV>"
  Bus Selector1/1 -> Sum/1  "<QV>"
  Bus Selector1/2 -> Sum1/1  "<QT>"
  Bus Selector/3 -> "Scalar2Bus "/3(A)  "<A_v>"
  "Scalar2Bus "/1(CoCl) -> CoCl/1
  Sum2/1 -> "Scalar2Bus "/4(CC)
  Bus Selector1/3 -> Sum2/1  "<CC>"
  Heater/1 -> Sum/2
  Bus Selector/2 -> Sum1/2  "<QT>"

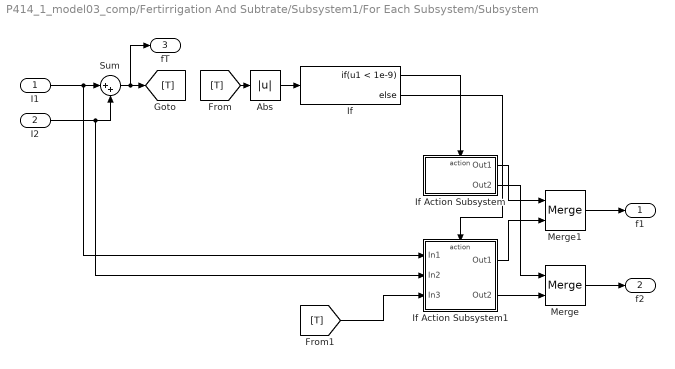
== system P414_1_model03_comp/Fertirrigation And Subtrate/Subsystem1/For Each Subsystem/Subsystem ==
  I1 : Inport
  I2 : Inport  Port=2
  Abs : Abs  ZeroCross=off
  If : If  IfExpression=u1 < 1e-9  ZeroCross=off
  If Action Subsystem : Subsystem  TreatAsAtomicUnit=on
  If Action Subsystem1 : Subsystem  TreatAsAtomicUnit=on
  Merge : Merge
  Merge1 : Merge
  Sum : Sum  Inputs=|++
  f1 : Outport
  f2 : Outport  Port=2
  fT : Outport  Port=3
  wires:
  I1/1 -> If Action Subsystem1/1(In1), Sum/1
  I2/1 -> If Action Subsystem1/2(In2), Sum/2
  Sum/1 -> fT/1, [T]
  If/1 -> If Action Subsystem/Action
  If/2 -> If Action Subsystem1/Action
  [T] -> If Action Subsystem1/3(In3)
  If Action Subsystem/2(Out2) -> Merge/1
  If Action Subsystem1/2(Out2) -> Merge/2
  Merge/1 -> f2/1
  Merge1/1 -> f1/1
  If Action Subsystem1/1(Out1) -> Merge1/2
  If Action Subsystem/1(Out1) -> Merge1/1
  Abs/1 -> If/1
  [T] -> Abs/1

== system P414_1_model03_comp/Fertirrigation And Subtrate/Subsystem1/Subsystem/If Action Subsystem ==
  Action Port : ActionPort  ActionPortLabel=if(u1 < 1e-9)
  Constant : Constant  Value=0
  Constant1 : Constant  Value=0
  Out1 : Outport
  Out2 : Outport  Port=2
  wires:
  Constant/1 -> Out1/1
  Constant1/1 -> Out2/1

== system P414_1_model03_comp/Fertirrigation And Subtrate/Subsystem1/Subsystem/If Action Subsystem1 ==
  In1 : Inport
  In2 : Inport  Port=2
  In3 : Inport  Port=3
  Action Port : ActionPort  ActionPortLabel=else
  Divide : Product  Inputs=*/
  Divide1 : Product  Inputs=*/
  Out1 : Outport
  Out2 : Outport  Port=2
  wires:
  In1/1 -> Divide/1
  In2/1 -> Divide1/1
  In3/1 -> Divide1/2, Divide/2
  Divide/1 -> Out1/1
  Divide1/1 -> Out2/1

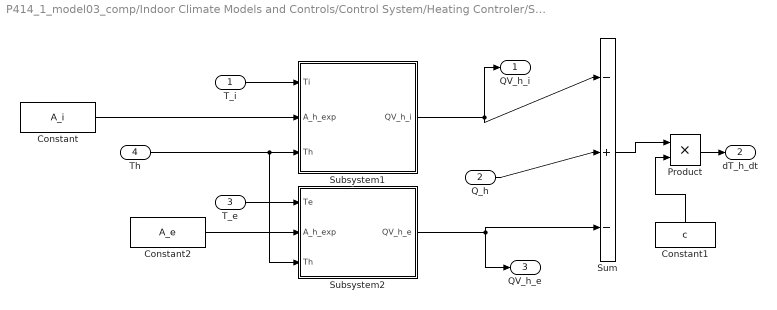
== system P414_1_model03_comp/Indoor Climate Models and Controls/Control System/Heating Controler/Subsystem ==
  T_i : Inport
  Q_h : Inport  Port=2
  T_e : Inport  Port=3
  Th : Inport  Port=4
  Constant : Constant  Value=A_i
  Constant1 : Constant  Value=c
  Constant2 : Constant  Value=A_e
  Product : Product
  Subsystem1 : Subsystem
  Subsystem2 : Subsystem
  Sum : Sum  Inputs=|-+-
  QV_h_i : Outport
  dT_h_dt : Outport  Port=2
  QV_h_e : Outport  Port=3
  wires:
  T_i/1 -> Subsystem1/1(Ti)
  Constant/1 -> Subsystem1/2(A_h_exp)
  Th/1 -> Subsystem2/3(Th), Subsystem1/3(Th)
  T_e/1 -> Subsystem2/1(Te)
  Subsystem1/1(QV_h_i) -> QV_h_i/1, Sum/1
  Subsystem2/1(QV_h_e) -> QV_h_e/1, Sum/3
  Q_h/1 -> Sum/2
  Sum/1 -> Product/1
  Constant1/1 -> Product/2
  Product/1 -> dT_h_dt/1
  Constant2/1 -> Subsystem2/2(A_h_exp)

== system P414_1_model03_comp/Indoor Climate Models and Controls/Control System/Heating Controler/Subsystem2 ==
  " Min" : Inport
  Max : Inport  Port=2
  T : Inport  Port=3
  If : If  NumInputs=3  IfExpression=u2 > u1  ElseIfExpressions=u2 < u3
  If Action Subsystem : Subsystem  TreatAsAtomicUnit=on
  If Action Subsystem1 : Subsystem  TreatAsAtomicUnit=on
  If Action Subsystem2 : Subsystem  TreatAsAtomicUnit=on
  Memory : Memory
  Merge : Merge  Inputs=3
  y : Outport
  wires:
  Memory/1 -> If Action Subsystem2/1(In1)
  Merge/1 -> y/1, Memory/1
  If Action Subsystem/1(Out1) -> Merge/1
  If Action Subsystem1/1(Out1) -> Merge/2
  If Action Subsystem2/1(Out1) -> Merge/3
  If/3 -> If Action Subsystem2/Action
  If/2 -> If Action Subsystem1/Action
  If/1 -> If Action Subsystem/Action
  Max/1 -> If/1
  " Min"/1 -> If/3
  T/1 -> If/2

== system P414_1_model03_comp/Indoor Climate Models and Controls/Control System/Selector/If Action Subsystem ==
  Windows : Inport
  Action Port : ActionPort  ActionPortLabel=else
  Constant2 : Constant  Value=WinAR
  Windows Connector : HORTISIM/Other  Functions/Windows Connector  SystemSampleTime=-1  VariantActivationTime=update diagram  Latency=0  AutoFrameSizeCalculation=off
      settings: SourceProductName=Horti Simulator
  Out1 : Outport
  wires:
  Windows/1 -> Windows Connector/1
  Constant2/1 -> Windows Connector/2
  Windows Connector/1 -> Out1/1

== system P414_1_model03_comp/Indoor Climate Models and Controls/Control System/Selector/If Action Subsystem1 ==
  In1 : Inport
  Action Port : ActionPort  ActionPortLabel=if(u2 > u1)
  Constant : Constant  Value=20 + 273.15
  Constant1 : Constant  Value=18 + 273.15
  Constant2 : Constant  Value=80
  Constant3 : Constant  Value=90
  Windows Controler : HORTISIM/Climate/Controls/Windows Controler  Power=100  max_night=max_night  tau=tau_win  RadThreshold=10  AR=WinAR
      settings: SourceProductName=Horti Simulator
  Out1 : Outport
  wires:
  Windows Controler/1 -> Out1/1  "Windows"
  Windows Controler/2 -> ?
  In1/1 -> Windows Controler/1
  Constant/1 -> Windows Controler/3
  Constant1/1 -> Windows Controler/2
  Constant2/1 -> Windows Controler/4
  Constant3/1 -> Windows Controler/5

== system P414_1_model03_comp/Indoor Climate Models and Controls/Control System/Subsystem/Scalar2Bus  ==
  QV : Inport
  QT : Inport  Port=2
  A : Inport  Port=3
  CC : Inport  Port=4
  Bus Creator : BusCreator  Inputs=4
  CoCl : Outport
  wires:
  A/1 -> Bus Creator/3  "A"
  CC/1 -> Bus Creator/4  "CC"
  QV/1 -> Bus Creator/1  "QV"
  Bus Creator/1 -> CoCl/1
  QT/1 -> Bus Creator/2  "QT"

== system P414_1_model03_comp/Fertirrigation And Subtrate/Subsystem1/For Each Subsystem/Subsystem/If Action Subsystem ==
  Action Port : ActionPort  ActionPortLabel=if(u1 < 1e-9)
  Constant : Constant  Value=0
  Constant1 : Constant  Value=0
  Out1 : Outport
  Out2 : Outport  Port=2
  wires:
  Constant/1 -> Out1/1
  Constant1/1 -> Out2/1

== system P414_1_model03_comp/Fertirrigation And Subtrate/Subsystem1/For Each Subsystem/Subsystem/If Action Subsystem1 ==
  In1 : Inport
  In2 : Inport  Port=2
  In3 : Inport  Port=3
  Action Port : ActionPort  ActionPortLabel=else
  Divide : Product  Inputs=*/
  Divide1 : Product  Inputs=*/
  Out1 : Outport
  Out2 : Outport  Port=2
  wires:
  In1/1 -> Divide/1
  In2/1 -> Divide1/1
  In3/1 -> Divide1/2, Divide/2
  Divide/1 -> Out1/1
  Divide1/1 -> Out2/1

== system P414_1_model03_comp/Indoor Climate Models and Controls/Control System/Heating Controler/Subsystem/Subsystem1 ==
  Ti : Inport
  A_h_exp : Inport  Port=2
  Th : Inport  Port=3
  Divide2 : Product  Inputs=****/
  Subsystem : Subsystem
  d_h1 : Constant  Value=1.5
  lambda thermal conductivity of air [W/m/K] : Constant  Value=0.025
  QV_h_i : Outport
  wires:
  Divide2/1 -> QV_h_i/1
  Subsystem/2(dT) -> Divide2/4
  Subsystem/1(Gr) -> Divide2/2
  d_h1/1 -> Divide2/5
  A_h_exp/1 -> Divide2/3
  lambda thermal conductivity of air [W/m/K]/1 -> Divide2/1
  Th/1 -> Subsystem/2(Th)
  Ti/1 -> Subsystem/1(Ti)

== system P414_1_model03_comp/Indoor Climate Models and Controls/Control System/Heating Controler/Subsystem/Subsystem2 ==
  Te : Inport
  A_h_exp : Inport  Port=2
  Th : Inport  Port=3
  Divide2 : Product  Inputs=****/
  Subsystem : Subsystem
  d_h1 : Constant  Value=1.5
  lambda thermal conductivity of air [W/m/K] : Constant  Value=0.025
  QV_h_e : Outport
  wires:
  Divide2/1 -> QV_h_e/1
  Subsystem/2(dT) -> Divide2/4
  Subsystem/1(Gr) -> Divide2/2
  d_h1/1 -> Divide2/5
  A_h_exp/1 -> Divide2/3
  lambda thermal conductivity of air [W/m/K]/1 -> Divide2/1
  Th/1 -> Subsystem/2(Th)
  Te/1 -> Subsystem/1(Ti)

== system P414_1_model03_comp/Indoor Climate Models and Controls/Control System/Heating Controler/Subsystem2/If Action Subsystem ==
  Action Port : ActionPort  ActionPortLabel=if(u2 > u1)
  Constant : Constant  Value=0
  Out1 : Outport
  wires:
  Constant/1 -> Out1/1

== system P414_1_model03_comp/Indoor Climate Models and Controls/Control System/Heating Controler/Subsystem2/If Action Subsystem1 ==
  Action Port : ActionPort  ActionPortLabel=elseif(u2 < u3)
  Constant : Constant
  Out1 : Outport
  wires:
  Constant/1 -> Out1/1

== system P414_1_model03_comp/Indoor Climate Models and Controls/Control System/Heating Controler/Subsystem2/If Action Subsystem2 ==
  In1 : Inport
  Action Port : ActionPort  ActionPortLabel=else
  Out1 : Outport
  wires:
  In1/1 -> Out1/1

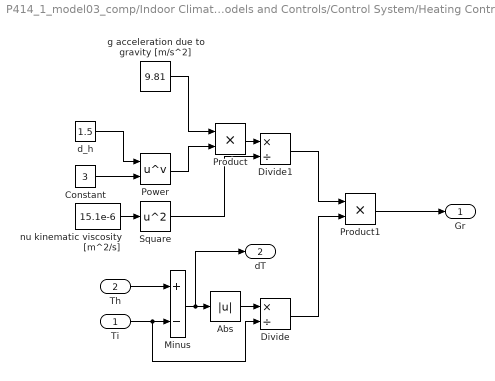
== system P414_1_model03_comp/Indoor Climate Models and Controls/Control System/Heating Controler/Subsystem/Subsystem1/Subsystem ==
  Ti : Inport
  Th : Inport  Port=2
  " nu kinematic viscosity [m^2/s]" : Constant  Value=15.1e-6
  Abs : Abs
  Constant : Constant  Value=3
  Divide : Product  Inputs=*/
  Divide1 : Product  Inputs=*/
  Minus : Sum  Inputs=+-
  Power : Math  Operator=pow  SaturateOnIntegerOverflow=on
  Product : Product
  Product1 : Product
  Square : Math  Operator=square  SaturateOnIntegerOverflow=on
  d_h : Constant  Value=1.5
  g acceleration due to gravity [m/s^2] : Constant  Value=9.81
  Gr : Outport
  dT : Outport  Port=2
  wires:
  g acceleration due to gravity [m/s^2]/1 -> Product/1
  Abs/1 -> Divide/1
  Divide1/1 -> Product1/1
  Divide/1 -> Product1/2
  Product1/1 -> Gr/1
  Square/1 -> Divide1/2
  Product/1 -> Divide1/1
  Constant/1 -> Power/2
  Th/1 -> Minus/1
  " nu kinematic viscosity [m^2/s]"/1 -> Square/1
  Minus/1 -> dT/1, Abs/1
  d_h/1 -> Power/1
  Power/1 -> Product/2
  Ti/1 -> Divide/2, Minus/2

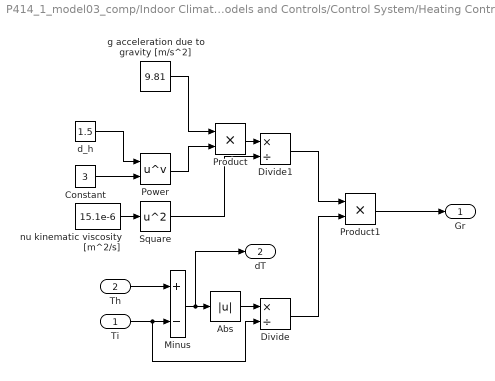
== system P414_1_model03_comp/Indoor Climate Models and Controls/Control System/Heating Controler/Subsystem/Subsystem2/Subsystem ==
  Ti : Inport
  Th : Inport  Port=2
  " nu kinematic viscosity [m^2/s]" : Constant  Value=15.1e-6
  Abs : Abs
  Constant : Constant  Value=3
  Divide : Product  Inputs=*/
  Divide1 : Product  Inputs=*/
  Minus : Sum  Inputs=+-
  Power : Math  Operator=pow  SaturateOnIntegerOverflow=on
  Product : Product
  Product1 : Product
  Square : Math  Operator=square  SaturateOnIntegerOverflow=on
  d_h : Constant  Value=1.5
  g acceleration due to gravity [m/s^2] : Constant  Value=9.81
  Gr : Outport
  dT : Outport  Port=2
  wires:
  g acceleration due to gravity [m/s^2]/1 -> Product/1
  Abs/1 -> Divide/1
  Divide1/1 -> Product1/1
  Divide/1 -> Product1/2
  Product1/1 -> Gr/1
  Square/1 -> Divide1/2
  Product/1 -> Divide1/1
  Constant/1 -> Power/2
  Th/1 -> Minus/1
  " nu kinematic viscosity [m^2/s]"/1 -> Square/1
  Minus/1 -> dT/1, Abs/1
  d_h/1 -> Power/1
  Power/1 -> Product/2
  Ti/1 -> Divide/2, Minus/2
